simulink model "modeloPlanta"  (R2018a)
settings: Solver=VariableStepAuto  StartTime=0.0  StopTime=100  RelTol=1e-3
values from neighbouring files (symbols this model uses):
  C = 2267    [params.m]    (also in paramsLinealizado.m)
  H_l = 1.05    [params.m]    (also in paramsLinealizado.m)
  n0_S = 1322    [params.m]    (also in paramsLinealizado.m)
  P_cp = 1924    [params.m]    (also in paramsLinealizado.m)
  Tinit = 260    [params.m]    (also in paramsLinealizado.m)
libraries: simulink x2
settings Model: Creator=wenap  LastModifiedBy=chris
settings DataIOCC: ReturnWorkspaceOutputs=on
settings SFSimCC: SimUseLocalCustomCode=on
settings RTWCC: RTWUseLocalCustomCode=on

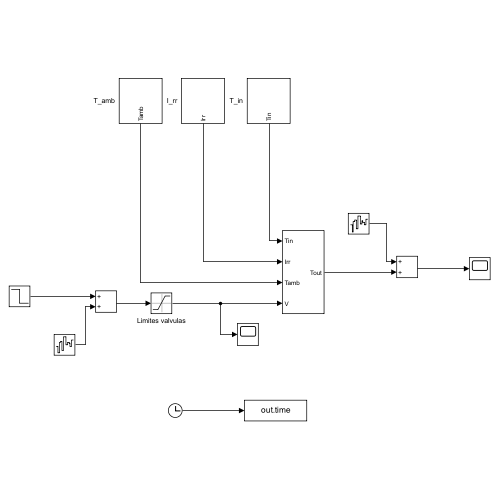
[thumbnail: Simulink's stored preview of the top-level diagram]
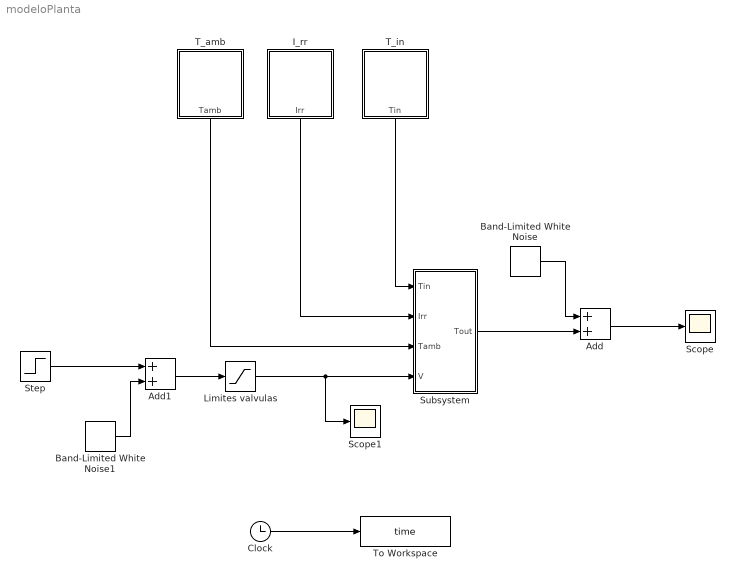
== system modeloPlanta ==
  Add : Sum
  Add1 : Sum
  Band-Limited White Noise : simulink/Sources/Band-Limited White Noise  Cov=[0.0001]  Ts=0.57  seed=[23341]
  Band-Limited White Noise1 : simulink/Sources/Band-Limited White Noise  Cov=[0.0001]  Ts=0.57  seed=[0]
  Clock : Clock
  I_rr : Subsystem
  Limites valvulas : Saturate  UpperLimit=12  LowerLimit=2
  Scope : Scope
  Scope1 : Scope
  Step : Step  Time=39  Before=8  After=7  SampleTime=0
  Subsystem : Subsystem
  T_amb : Subsystem
  T_in : Subsystem
  To Workspace : ToWorkspace  VariableName=time  SampleTime=-1
  wires:
  T_in/1(Tin) -> Subsystem/1(Tin)
  I_rr/1(Irr) -> Subsystem/2(Irr)
  T_amb/1(Tamb) -> Subsystem/3(Tamb)
  Add/1 -> Scope/1
  Subsystem/1(Tout) -> Add/2
  Band-Limited White Noise/1 -> Add/1
  Band-Limited White Noise1/1 -> Add1/2
  Limites valvulas/1 -> Scope1/1, Subsystem/4(V)
  Step/1 -> Add1/1
  Add1/1 -> Limites valvulas/1
  Clock/1 -> To Workspace/1

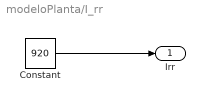
== system modeloPlanta/I_rr ==
  Constant : Constant  Value=920
  Irr : Outport
  wires:
  Constant/1 -> Irr/1

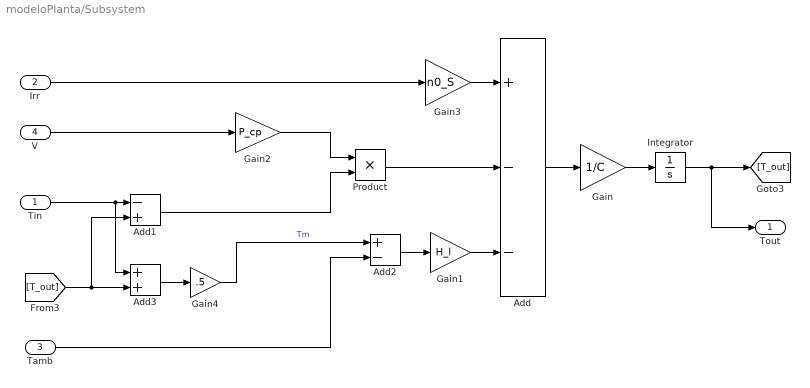
== system modeloPlanta/Subsystem ==
  Tin : Inport
  Irr : Inport  Port=2
  Tamb : Inport  Port=3
  V : Inport  Port=4
  Add : Sum  Inputs=+--
  Add1 : Sum  Inputs=-+
  Add2 : Sum  Inputs=+-
  Add3 : Sum
  Gain : Gain  Gain=1/C
  Gain1 : Gain  Gain=H_l
  Gain2 : Gain  Gain=P_cp
  Gain3 : Gain  Gain=n0_S
  Gain4 : Gain  Gain=.5
  Integrator : Integrator  InitialCondition=Tinit
  Product : Product
  Tout : Outport
  wires:
  Gain2/1 -> Product/1
  Gain3/1 -> Add/1
  Add2/1 -> Gain1/1
  Add1/1 -> Product/2
  Gain/1 -> Integrator/1
  Integrator/1 -> Tout/1, [T_out]
  Add3/1 -> Gain4/1
  Tamb/1 -> Add2/2
  [T_out] -> Add3/2, Add1/2
  Tin/1 -> Add3/1, Add1/1
  Add/1 -> Gain/1
  Product/1 -> Add/2
  Gain1/1 -> Add/3
  Irr/1 -> Gain3/1
  Gain4/1 -> Add2/1  "Tm"
  V/1 -> Gain2/1

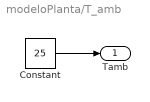
== system modeloPlanta/T_amb ==
  Constant : Constant  Value=25
  Tamb : Outport
  wires:
  Constant/1 -> Tamb/1

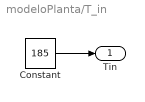
== system modeloPlanta/T_in ==
  Constant : Constant  Value=185
  Tin : Outport
  wires:
  Constant/1 -> Tin/1
